simulink model "CVS_Model"  (R2021a)
settings: Solver=VariableStepAuto  StartTime=0.0  StopTime=2.4  RelTol=1e-3
libraries: ee_lib x804, fl_lib x456, nesl_utility x48, simulink x4
(part 8 of 8)

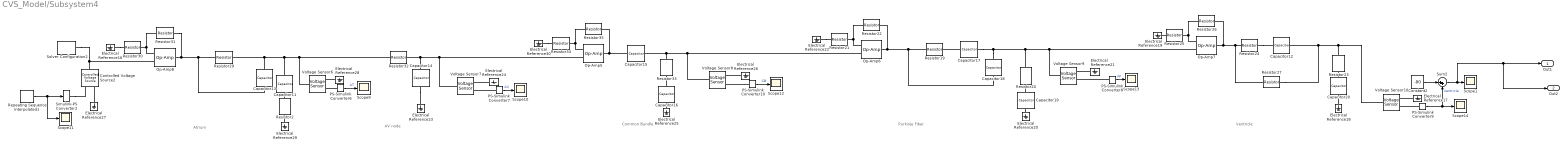
== system CVS_Model/Subsystem4 ==
  note: Atrium
  note: Common Bundle
  note: Ventricle
  note: AV node
  note: Purkinje Fiber
  Capacitor11 : fl_lib/Electrical/Electrical Elements/Capacitor  c=80 uF  r=0 Ohm  g=0 1/Ohm  i_specify=off  i_priority=None  i=0 A  i_nominal_specify=off  i_nominal_unit=A  i_nominal_value=1  v_specify=off  v_priority=None  v=0 V  v_nominal_specify=off  v_nominal_unit=V  v_nominal_value=1  vc_specify=off  vc_priority=High  vc=0 V  vc_nominal_specify=off  vc_nominal_unit=V  vc_nominal_value=1
  Capacitor12 : fl_lib/Electrical/Electrical Elements/Capacitor  c=8 uF  r=0 Ohm  g=0 1/Ohm  i_specify=off  i_priority=None  i=0 A  i_nominal_specify=off  i_nominal_unit=A  i_nominal_value=1  v_specify=off  v_priority=None  v=0 V  v_nominal_specify=off  v_nominal_unit=V  v_nominal_value=1  vc_specify=off  vc_priority=High  vc=0 V  vc_nominal_specify=off  vc_nominal_unit=V  vc_nominal_value=1
  Capacitor13 : fl_lib/Electrical/Electrical Elements/Capacitor  c=80 uF  r=0 Ohm  g=0 1/Ohm  i_specify=off  i_priority=None  i=0 A  i_nominal_specify=off  i_nominal_unit=A  i_nominal_value=1  v_specify=off  v_priority=None  v=0 V  v_nominal_specify=off  v_nominal_unit=V  v_nominal_value=1  vc_specify=off  vc_priority=High  vc=0 V  vc_nominal_specify=off  vc_nominal_unit=V  vc_nominal_value=1
  Capacitor14 : fl_lib/Electrical/Electrical Elements/Capacitor  c=20 uF  r=0 Ohm  g=0 1/Ohm  i_specify=off  i_priority=None  i=0 A  i_nominal_specify=off  i_nominal_unit=A  i_nominal_value=1  v_specify=off  v_priority=None  v=0 V  v_nominal_specify=off  v_nominal_unit=V  v_nominal_value=1  vc_specify=off  vc_priority=High  vc=0 V  vc_nominal_specify=off  vc_nominal_unit=V  vc_nominal_value=1
  Capacitor15 : fl_lib/Electrical/Electrical Elements/Capacitor  c=10 uF  r=1e-6 Ohm  g=0 1/Ohm  i_specify=off  i_priority=None  i=0 A  i_nominal_specify=off  i_nominal_unit=A  i_nominal_value=1  v_specify=off  v_priority=None  v=0 V  v_nominal_specify=off  v_nominal_unit=V  v_nominal_value=1  vc_specify=off  vc_priority=High  vc=0 V  vc_nominal_specify=off  vc_nominal_unit=V  vc_nominal_value=1
  Capacitor16 : fl_lib/Electrical/Electrical Elements/Capacitor  c=12 uF  r=0 Ohm  g=0 1/Ohm  i_specify=off  i_priority=None  i=0 A  i_nominal_specify=off  i_nominal_unit=A  i_nominal_value=1  v_specify=off  v_priority=None  v=0 V  v_nominal_specify=off  v_nominal_unit=V  v_nominal_value=1  vc_specify=off  vc_priority=High  vc=0 V  vc_nominal_specify=off  vc_nominal_unit=V  vc_nominal_value=1
  Capacitor17 : fl_lib/Electrical/Electrical Elements/Capacitor  c=20 uF  r=1e-6 Ohm  g=0 1/Ohm  i_specify=off  i_priority=None  i=0 A  i_nominal_specify=off  i_nominal_unit=A  i_nominal_value=1  v_specify=off  v_priority=None  v=0 V  v_nominal_specify=off  v_nominal_unit=V  v_nominal_value=1  vc_specify=off  vc_priority=High  vc=0 V  vc_nominal_specify=off  vc_nominal_unit=V  vc_nominal_value=1
  Capacitor18 : fl_lib/Electrical/Electrical Elements/Capacitor  c=30 uF  r=1e-6 Ohm  g=0 1/Ohm  i_specify=off  i_priority=None  i=0 A  i_nominal_specify=off  i_nominal_unit=A  i_nominal_value=1  v_specify=off  v_priority=None  v=0 V  v_nominal_specify=off  v_nominal_unit=V  v_nominal_value=1  vc_specify=off  vc_priority=High  vc=0 V  vc_nominal_specify=off  vc_nominal_unit=V  vc_nominal_value=1
  Capacitor19 : fl_lib/Electrical/Electrical Elements/Capacitor  c=50 uF  r=1e-6 Ohm  g=0 1/Ohm  i_specify=off  i_priority=None  i=0 A  i_nominal_specify=off  i_nominal_unit=A  i_nominal_value=1  v_specify=off  v_priority=None  v=0 V  v_nominal_specify=off  v_nominal_unit=V  v_nominal_value=1  vc_specify=off  vc_priority=High  vc=0 V  vc_nominal_specify=off  vc_nominal_unit=V  vc_nominal_value=1
  Capacitor20 : fl_lib/Electrical/Electrical Elements/Capacitor  c=2.5 uF  r=0 Ohm  g=0 1/Ohm  i_specify=off  i_priority=None  i=0 A  i_nominal_specify=off  i_nominal_unit=A  i_nominal_value=1  v_specify=off  v_priority=None  v=0 V  v_nominal_specify=off  v_nominal_unit=V  v_nominal_value=1  vc_specify=off  vc_priority=High  vc=0 V  vc_nominal_specify=off  vc_nominal_unit=V  vc_nominal_value=1
  Constant2 : Constant  Value=-80
  Controlled Voltage Source2 : fl_lib/Electrical/Electrical Sources/Controlled Voltage Source
  Electrical Reference{16..30} (15 alike) : fl_lib/Electrical/Electrical Elements/Electrical Reference
  Op-Amp{5..8} (4 alike) : fl_lib/Electrical/Electrical Elements/Op-Amp  outI_specify=off  outI_priority=None  outI=0 A  outI_nominal_specify=off  outI_nominal_unit=A  outI_nominal_value=1
  PS-Simulink Converter{6..10} (5 alike) : nesl_utility/PS-Simulink Converter  PhysicalDomain=network_engine_domain  SubClassName=ps_output  LeftPortType=input  RightPortType=output  PseudoPeriodic=off  Frequencies=[]  Unit=inherit  AffineConversion=off
      settings: SourceProductBaseCode=PW,SS
  Repeating Sequence Interpolated1 : simulink/Sources/Repeating Sequence Interpolated  OutValues=[0 0.01 60 -3 0].'  TimeValues=[0 0.1 0.12 0.4 0.8].'  LookUpMeth=Interpolation-Use End Values  tsamp=0.0001  OutMin=[]  OutMax=[]  OutDataTypeStr=double  OutputDataTypeScalingMode=double  OutDataType=fixdt(0,8)  OutScaling=2^-10
  Resistor19 : fl_lib/Electrical/Electrical Elements/Resistor  R=0.2 kOhm  i_specify=off  i_priority=None  i=0 A  i_nominal_specify=off  i_nominal_unit=A  i_nominal_value=1  v_specify=off  v_priority=None  v=0 V  v_nominal_specify=off  v_nominal_unit=V  v_nominal_value=1
  Resistor2 : fl_lib/Electrical/Electrical Elements/Resistor  R=0.4 kOhm  i_specify=off  i_priority=None  i=0 A  i_nominal_specify=off  i_nominal_unit=A  i_nominal_value=1  v_specify=off  v_priority=None  v=0 V  v_nominal_specify=off  v_nominal_unit=V  v_nominal_value=1
  Resistor20 : fl_lib/Electrical/Electrical Elements/Resistor  R=0.4 kOhm  i_specify=off  i_priority=None  i=0 A  i_nominal_specify=off  i_nominal_unit=A  i_nominal_value=1  v_specify=off  v_priority=None  v=0 V  v_nominal_specify=off  v_nominal_unit=V  v_nominal_value=1
  Resistor21 : fl_lib/Electrical/Electrical Elements/Resistor  R=0.7 kOhm  i_specify=off  i_priority=None  i=0 A  i_nominal_specify=off  i_nominal_unit=A  i_nominal_value=1  v_specify=off  v_priority=None  v=0 V  v_nominal_specify=off  v_nominal_unit=V  v_nominal_value=1
  Resistor{22,26,31,35} (4 alike) : fl_lib/Electrical/Electrical Elements/Resistor  R=1.5 kOhm  i_specify=off  i_priority=None  i=0 A  i_nominal_specify=off  i_nominal_unit=A  i_nominal_value=1  v_specify=off  v_priority=None  v=0 V  v_nominal_specify=off  v_nominal_unit=V  v_nominal_value=1
  Resistor23 : fl_lib/Electrical/Electrical Elements/Resistor  R=1 kOhm  i_specify=off  i_priority=None  i=0 A  i_nominal_specify=off  i_nominal_unit=A  i_nominal_value=1  v_specify=off  v_priority=None  v=0 V  v_nominal_specify=off  v_nominal_unit=V  v_nominal_value=1
  Resistor24 : fl_lib/Electrical/Electrical Elements/Resistor  R=0.5 kOhm  i_specify=off  i_priority=None  i=0 A  i_nominal_specify=off  i_nominal_unit=A  i_nominal_value=1  v_specify=off  v_priority=None  v=0 V  v_nominal_specify=off  v_nominal_unit=V  v_nominal_value=1
  Resistor25 : fl_lib/Electrical/Electrical Elements/Resistor  R=3.5 kOhm  i_specify=off  i_priority=None  i=0 A  i_nominal_specify=off  i_nominal_unit=A  i_nominal_value=1  v_specify=off  v_priority=None  v=0 V  v_nominal_specify=off  v_nominal_unit=V  v_nominal_value=1
  Resistor27 : fl_lib/Electrical/Electrical Elements/Resistor  R=2.5 kOhm  i_specify=off  i_priority=None  i=0 A  i_nominal_specify=off  i_nominal_unit=A  i_nominal_value=1  v_specify=off  v_priority=None  v=0 V  v_nominal_specify=off  v_nominal_unit=V  v_nominal_value=1
  Resistor29 : fl_lib/Electrical/Electrical Elements/Resistor  R=0.3 kOhm  i_specify=off  i_priority=None  i=0 A  i_nominal_specify=off  i_nominal_unit=A  i_nominal_value=1  v_specify=off  v_priority=None  v=0 V  v_nominal_specify=off  v_nominal_unit=V  v_nominal_value=1
  Resistor30 : fl_lib/Electrical/Electrical Elements/Resistor  R=2 kOhm  i_specify=off  i_priority=None  i=0 A  i_nominal_specify=off  i_nominal_unit=A  i_nominal_value=1  v_specify=off  v_priority=None  v=0 V  v_nominal_specify=off  v_nominal_unit=V  v_nominal_value=1
  Resistor32 : fl_lib/Electrical/Electrical Elements/Resistor  R=0.4 kOhm  i_specify=off  i_priority=None  i=0 A  i_nominal_specify=off  i_nominal_unit=A  i_nominal_value=1  v_specify=off  v_priority=None  v=0 V  v_nominal_specify=off  v_nominal_unit=V  v_nominal_value=1
  Resistor33 : fl_lib/Electrical/Electrical Elements/Resistor  R=0.5 kOhm  i_specify=off  i_priority=None  i=0 A  i_nominal_specify=off  i_nominal_unit=A  i_nominal_value=1  v_specify=off  v_priority=None  v=0 V  v_nominal_specify=off  v_nominal_unit=V  v_nominal_value=1
  Resistor34 : fl_lib/Electrical/Electrical Elements/Resistor  R=2 kOhm  i_specify=off  i_priority=None  i=0 A  i_nominal_specify=off  i_nominal_unit=A  i_nominal_value=1  v_specify=off  v_priority=None  v=0 V  v_nominal_specify=off  v_nominal_unit=V  v_nominal_value=1
  Scope{1,9..14} (7 alike) : Scope
  Simulink-PS Converter2 : nesl_utility/Simulink-PS Converter  PhysicalDomain=network_engine_domain  SubClassName=ps_input  LeftPortType=input  RightPortType=output  PseudoPeriodic=off  Frequencies=[]  NoiseDistribution=none  NoiseParameters=[]  Unit=1  AffineConversion=off  FilteringAndDerivatives=provide  SimscapeFilterOrder=1  InputFilterTimeConstant=0.001  UdotUserProvided=0
      settings: SourceProductBaseCode=PW,SS
  Solver Configuration2 : nesl_utility/Solver Configuration  PhysicalDomain=network_engine_domain  SubClassName=solver  LeftPortType=input  RightPortType=generic  Tones=[]  Harmonics=[]  SimulateNoise=off  Profile=off  UseLocalSampling=off  EnableSwitchedLinearOptims=on  FrequencyDomain=off  UseCCode=off  RelTol=0.001  AbsTol=1e-06  MinStep=1e-09  ToWorkspace=off  RevertToSquareIcSolve=off  NumHomotopyIterations=100  PhasorMode=off  PhasorModeNumHarmonics=1  DoDC=off  ResidualTolerance=1e-09  UseLocalSolver=off  LocalSolverChoice=NE_BACKWARD_EULER_ADVANCER  LocalSolverSampleTime=0.001  DoFixedCost=off  MaxNonlinIter=3  MaxModeIter=2  ComputeImpulses=off  ImpulseIterations=2  LinearAlgebra=auto  EquationFormulation=NE_TIME_EF  DelaysMemoryBudget=1024  AutomaticFiltering=on  FilteringTimeConstant=0.001  PartitionStorageMethod=AS_NEEDED  PartitionMemoryBudget=1024  PartitionMethod=ROBUST
      settings: SourceProductBaseCode=PW,SS
  Sum2 : Sum  Inputs=|++
  Voltage Sensor{6..10} (5 alike) : fl_lib/Electrical/Electrical Sensors/Voltage Sensor
  Out1 : Outport
  Out2 : Outport  Port=2
  wires:
  PS-Simulink Converter8/1 -> Scope13/1  "PF"
  Repeating Sequence Interpolated1/1 -> Simulink-PS Converter2/1, Scope11/1
  Sum2/1 -> Out2/1, Out1/1, Scope1/1
  PS-Simulink Converter10/1 -> Scope12/1  "CB"
  Constant2/1 -> Sum2/1
  PS-Simulink Converter9/1 -> Scope14/1, Sum2/2  "Ventricle"
  PS-Simulink Converter7/1 -> Scope10/1  "AV"
  PS-Simulink Converter6/1 -> Scope9/1  "AT"
  connections:
  Op-Amp6/LConn1 -- Voltage Sensor8/LConn1 -- Resistor33/LConn1 -- Capacitor15/RConn1
  Resistor27/LConn1 -- Capacitor12/RConn1 -- Resistor23/LConn1 -- Voltage Sensor10/LConn1
  Resistor34/RConn1 -- Op-Amp5/LConn2 -- Resistor35/LConn1
  Op-Amp5/RConn1 -- Resistor35/RConn1 -- Capacitor15/LConn1
  Resistor29/RConn1 -- Capacitor13/LConn1 -- Capacitor11/LConn1 -- Voltage Sensor6/LConn1 -- Resistor32/LConn1
  Capacitor18/LConn1 -- Capacitor17/RConn1 -- Resistor20/LConn1 -- Voltage Sensor9/LConn1 -- Op-Amp7/LConn1
  Resistor25/RConn1 -- Op-Amp7/LConn2 -- Resistor26/LConn1
  Solver Configuration2/RConn1 -- Op-Amp8/LConn1 -- Controlled Voltage Source2/LConn1
  Resistor32/RConn1 -- Capacitor14/LConn1 -- Op-Amp5/LConn1 -- Voltage Sensor7/LConn1
  Resistor30/RConn1 -- Op-Amp8/LConn2 -- Resistor31/LConn1
  Resistor21/RConn1 -- Op-Amp6/LConn2 -- Resistor22/LConn1
  Op-Amp6/RConn1 -- Capacitor18/RConn1 -- Resistor19/LConn1 -- Resistor22/RConn1
  Resistor26/RConn1 -- Op-Amp7/RConn1 -- Resistor24/LConn1 -- Resistor27/RConn1
  Electrical Reference21/LConn1 -- Voltage Sensor9/RConn2
  Simulink-PS Converter2/RConn1 -- Controlled Voltage Source2/RConn1
  Electrical Reference16/LConn1 -- Resistor30/LConn1
  Electrical Reference17/LConn1 -- Voltage Sensor10/RConn2
  PS-Simulink Converter8/LConn1 -- Voltage Sensor9/RConn1
  Capacitor11/RConn1 -- Resistor2/LConn1
  Electrical Reference26/LConn1 -- Voltage Sensor8/RConn2
  Electrical Reference27/LConn1 -- Controlled Voltage Source2/RConn2
  Capacitor19/RConn1 -- Electrical Reference20/LConn1
  PS-Simulink Converter9/LConn1 -- Voltage Sensor10/RConn1
  Electrical Reference19/LConn1 -- Resistor25/LConn1
  PS-Simulink Converter6/LConn1 -- Voltage Sensor6/RConn1
  Electrical Reference30/LConn1 -- Resistor34/LConn1
  PS-Simulink Converter7/LConn1 -- Voltage Sensor7/RConn1
  Capacitor19/LConn1 -- Resistor20/RConn1
  PS-Simulink Converter10/LConn1 -- Voltage Sensor8/RConn1
  Resistor24/RConn1 -- Capacitor12/LConn1
  Electrical Reference24/LConn1 -- Voltage Sensor7/RConn2
  Capacitor14/RConn1 -- Electrical Reference23/LConn1
  Electrical Reference28/LConn1 -- Voltage Sensor6/RConn2
  Electrical Reference22/LConn1 -- Resistor21/LConn1
  Capacitor16/LConn1 -- Resistor33/RConn1
  Capacitor16/RConn1 -- Electrical Reference25/LConn1
  Resistor23/RConn1 -- Capacitor20/LConn1
  Electrical Reference18/LConn1 -- Capacitor20/RConn1
  Electrical Reference29/LConn1 -- Resistor2/RConn1
  Capacitor17/LConn1 -- Resistor19/RConn1
  Capacitor13/RConn1 -- Resistor29/LConn1 -- Resistor31/RConn1 -- Op-Amp8/RConn1
